simulink model "assignment_2_simulink_q13"  (R2023a)
settings: Solver=VariableStepAuto  StartTime=0.0  StopTime=0.5  MaxStep=1e-4  RelTol=1e-3
settings Model: Creator=chowd  LastModifiedBy=chowd
settings DataIOCC: ReturnWorkspaceOutputs=off

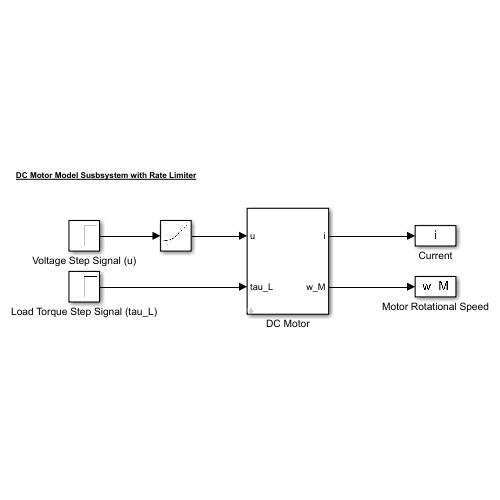
[thumbnail: Simulink's stored preview of the top-level diagram]
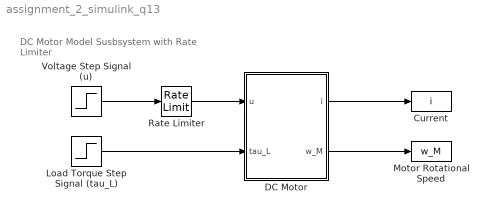
== system assignment_2_simulink_q13 ==
  note: DC Motor Model Susbsystem with Rate Limiter
  Current : ToWorkspace  VariableName=i  SaveFormat=Timeseries  SampleTime=-1
  DC Motor : Subsystem  mask{R=0.5, L=2.5e-3, k=0.35, J=1e-3}
      mask prompts: R "R (ohm)"; L "L (H)"; k "k (Vs)"; J "J (kgm^2)"
  Load Torque Step Signal (tau_L) : Step  Time=0.3  After=7  SampleTime=0.1
  Motor Rotational Speed : ToWorkspace  VariableName=w_M  SaveFormat=Timeseries  SampleTime=-1
  Rate Limiter : RateLimiter  RisingSlewLimit=120/0.1  FallingSlewLimit=-120/0.1  SampleTimeMode=inherited
  Voltage Step Signal (u) : Step  Time=0.1  After=120  SampleTime=T_sw/2  mask{T_sw=200e-6}
      mask prompts: T_sw "T_sw (s)"
  wires:
  DC Motor/1(i) -> Current/1
  DC Motor/2(w_M) -> Motor Rotational Speed/1
  Load Torque Step Signal (tau_L)/1 -> DC Motor/2(tau_L)
  Voltage Step Signal (u)/1 -> Rate Limiter/1
  Rate Limiter/1 -> DC Motor/1(u)

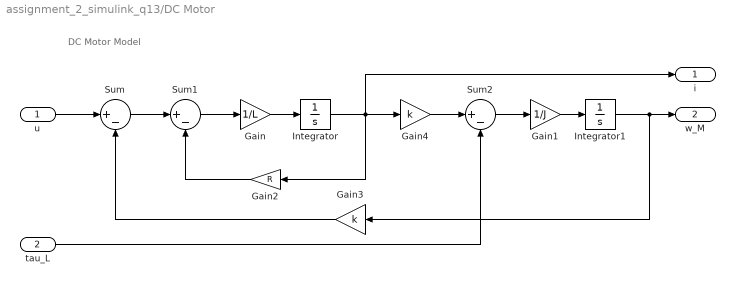
== system assignment_2_simulink_q13/DC Motor ==
  note: DC Motor Model
  u : Inport
  tau_L : Inport  Port=2
  Gain : Gain  Gain=1/L
  Gain1 : Gain  Gain=1/J
  Gain2 : Gain  Gain=R
  Gain3 : Gain  Gain=k
  Gain4 : Gain  Gain=k
  Integrator : Integrator
  Integrator1 : Integrator
  Sum : Sum  Inputs=|+-
  Sum1 : Sum  Inputs=|+-
  Sum2 : Sum  Inputs=|+-
  i : Outport
  w_M : Outport  Port=2
  wires:
  Gain/1 -> Integrator/1
  Sum2/1 -> Gain1/1
  Sum/1 -> Sum1/1
  u/1 -> Sum/1
  Integrator/1 -> Gain2/1, i/1, Gain4/1
  Sum1/1 -> Gain/1
  Gain2/1 -> Sum1/2
  Gain3/1 -> Sum/2
  tau_L/1 -> Sum2/2
  Integrator1/1 -> w_M/1, Gain3/1
  Gain4/1 -> Sum2/1
  Gain1/1 -> Integrator1/1
